simulink model "carsim_ekf_jonathan"  (R2024a)
settings: Solver=VariableStepAuto  StartTime=0.0  StopTime=40  RelTol=1e-3
model workspace (MAT data in the model file):
  Ts = 0.01
  a = 0.9
  b = 0.8
  for_ekf = mamfis
  for_ekf.Name = "for_ekf"
  for_ekf.Type = "mamdani"
  for_ekf.AndMethod = "min"
  for_ekf.OrMethod = "max"
  for_ekf.FuzzyInferenceSystem.LocalImplicationMethod = "min"
  for_ekf.FuzzyInferenceSystem.LocalAggregationMethod = "max"
  for_ekf.FuzzyInferenceSystem.LocalDefuzzificationMethod = "centroid"
  for_ekf.Inputs = fisvar
  for_ekf.Inputs.LocalName = "input1"
  for_ekf.Inputs.Range = [-30 30]
  for_ekf.Inputs.EvalfisData.name = ' '
  for_ekf.Inputs.EvalfisData.range = [-30 30]
  for_ekf.Inputs.EvalfisData.mf(1).name = ' '
  for_ekf.Inputs.EvalfisData.mf(1).type = 'linzmf'
  for_ekf.Inputs.EvalfisData.mf(1).params = [-20 -10]
  for_ekf.Inputs.EvalfisData.mf(2).name = ' '
  for_ekf.Inputs.EvalfisData.mf(2).type = 'trapmf'
  for_ekf.Inputs.EvalfisData.mf(2).params = [-20 -10 10 20]
  for_ekf.Inputs.EvalfisData.mf(3).name = ' '
  for_ekf.Inputs.EvalfisData.mf(3).type = 'linsmf'
  for_ekf.Inputs.EvalfisData.mf(3).params = [10 20]
  for_ekf.Inputs.LocalMembershipFunctions(1) = fismf
  for_ekf.Inputs.LocalMembershipFunctions(1).Function : function handle (value not decoded)
  for_ekf.Inputs.LocalMembershipFunctions(1).Parameters = [-20 -10]
  for_ekf.Inputs.LocalMembershipFunctions(1).ParameterValueValidator : function handle (value not decoded)
  for_ekf.Inputs.LocalMembershipFunctions(1).NumParameters = 2
  for_ekf.Inputs.LocalMembershipFunctions(1).TypeStr = "linzmf"
  for_ekf.Inputs.LocalMembershipFunctions(1).EvalfisData.name = ' '
  for_ekf.Inputs.LocalMembershipFunctions(1).EvalfisData.type = 'linzmf'
  for_ekf.Inputs.LocalMembershipFunctions(1).EvalfisData.params = [-20 -10]
  for_ekf.Inputs.LocalMembershipFunctions(1).fuzzy.internal.fis.MembershipFunction.LocalName = "high1"
  for_ekf.Inputs.LocalMembershipFunctions(1).UnmatchedInputArguments = struct()
  for_ekf.Inputs.LocalMembershipFunctions(2) = fismf
  for_ekf.Inputs.LocalMembershipFunctions(2).Function : function handle (value not decoded)
  for_ekf.Inputs.LocalMembershipFunctions(2).Parameters = [-20 -10 10 20]
  for_ekf.Inputs.LocalMembershipFunctions(2).ParameterValueValidator : function handle (value not decoded)
  for_ekf.Inputs.LocalMembershipFunctions(2).NumParameters = 4
  for_ekf.Inputs.LocalMembershipFunctions(2).TypeStr = "trapmf"
  for_ekf.Inputs.LocalMembershipFunctions(2).EvalfisData.name = ' '
  for_ekf.Inputs.LocalMembershipFunctions(2).EvalfisData.type = 'trapmf'
  for_ekf.Inputs.LocalMembershipFunctions(2).EvalfisData.params = [-20 -10 10 20]
  for_ekf.Inputs.LocalMembershipFunctions(2).fuzzy.internal.fis.MembershipFunction.LocalName = "mf2"
  for_ekf.Inputs.LocalMembershipFunctions(2).UnmatchedInputArguments = struct()
  for_ekf.Inputs.LocalMembershipFunctions(3) = fismf
  for_ekf.Inputs.LocalMembershipFunctions(3).Function : function handle (value not decoded)
  for_ekf.Inputs.LocalMembershipFunctions(3).Parameters = [10 20]
  for_ekf.Inputs.LocalMembershipFunctions(3).ParameterValueValidator : function handle (value not decoded)
  for_ekf.Inputs.LocalMembershipFunctions(3).NumParameters = 2
  for_ekf.Inputs.LocalMembershipFunctions(3).TypeStr = "linsmf"
  for_ekf.Inputs.LocalMembershipFunctions(3).EvalfisData.name = ' '
  for_ekf.Inputs.LocalMembershipFunctions(3).EvalfisData.type = 'linsmf'
  for_ekf.Inputs.LocalMembershipFunctions(3).EvalfisData.params = [10 20]
  for_ekf.Inputs.LocalMembershipFunctions(3).fuzzy.internal.fis.MembershipFunction.LocalName = "high2"
  for_ekf.Inputs.LocalMembershipFunctions(3).UnmatchedInputArguments = struct()
  for_ekf.Outputs = fisvar
  for_ekf.Outputs.LocalName = "output1"
  for_ekf.Outputs.Range = [0 10000]
  for_ekf.Outputs.EvalfisData.name = ' '
  for_ekf.Outputs.EvalfisData.range = [0 10000]
  for_ekf.Outputs.EvalfisData.mf(1).name = ' '
  for_ekf.Outputs.EvalfisData.mf(1).type = 'trimf'
  for_ekf.Outputs.EvalfisData.mf(1).params = [10000 10000 10000]
  for_ekf.Outputs.EvalfisData.mf(2).name = ' '
  for_ekf.Outputs.EvalfisData.mf(2).type = 'trimf'
  for_ekf.Outputs.EvalfisData.mf(2).params = [0 0 0]
  for_ekf.Outputs.LocalMembershipFunctions(1) = fismf
  for_ekf.Outputs.LocalMembershipFunctions(1).Function : function handle (value not decoded)
  for_ekf.Outputs.LocalMembershipFunctions(1).Parameters = [10000 10000 10000]
  for_ekf.Outputs.LocalMembershipFunctions(1).ParameterValueValidator : function handle (value not decoded)
  for_ekf.Outputs.LocalMembershipFunctions(1).NumParameters = 3
  for_ekf.Outputs.LocalMembershipFunctions(1).TypeStr = "trimf"
  for_ekf.Outputs.LocalMembershipFunctions(1).EvalfisData.name = ' '
  for_ekf.Outputs.LocalMembershipFunctions(1).EvalfisData.type = 'trimf'
  for_ekf.Outputs.LocalMembershipFunctions(1).EvalfisData.params = [10000 10000 10000]
  for_ekf.Outputs.LocalMembershipFunctions(1).fuzzy.internal.fis.MembershipFunction.LocalName = "mf1"
  for_ekf.Outputs.LocalMembershipFunctions(1).UnmatchedInputArguments = struct()
  for_ekf.Outputs.LocalMembershipFunctions(2) = fismf
  for_ekf.Outputs.LocalMembershipFunctions(2).Function : function handle (value not decoded)
  for_ekf.Outputs.LocalMembershipFunctions(2).Parameters = [0 0 0]
  for_ekf.Outputs.LocalMembershipFunctions(2).ParameterValueValidator : function handle (value not decoded)
  for_ekf.Outputs.LocalMembershipFunctions(2).NumParameters = 3
  for_ekf.Outputs.LocalMembershipFunctions(2).TypeStr = "trimf"
  for_ekf.Outputs.LocalMembershipFunctions(2).EvalfisData.name = ' '
  for_ekf.Outputs.LocalMembershipFunctions(2).EvalfisData.type = 'trimf'
  for_ekf.Outputs.LocalMembershipFunctions(2).EvalfisData.params = [0 0 0]
  for_ekf.Outputs.LocalMembershipFunctions(2).fuzzy.internal.fis.MembershipFunction.LocalName = "mf2"
  for_ekf.Outputs.LocalMembershipFunctions(2).UnmatchedInputArguments = struct()
  for_ekf.Rules(1) = fisrule
  for_ekf.Rules(1).LocalAntecedent = 1
  for_ekf.Rules(1).LocalConsequent = 1
  for_ekf.Rules(1).LocalDescription.input.name = "input1"
  for_ekf.Rules(1).LocalDescription.input.mf = "high1"
  for_ekf.Rules(1).LocalDescription.input.complement = 0
  for_ekf.Rules(1).LocalDescription.output.name = "output1"
  for_ekf.Rules(1).LocalDescription.output.mf = "mf1"
  for_ekf.Rules(1).LocalDescription.output.complement = 0
  for_ekf.Rules(1).LocalDescription.weight = 1
  for_ekf.Rules(1).LocalDescription.connection = 1
  for_ekf.Rules(1).LocalWeight = 1
  for_ekf.Rules(1).LocalConnection = 1
  for_ekf.Rules(1).EvalfisData.antecedent = 1
  for_ekf.Rules(1).EvalfisData.consequent = 1
  for_ekf.Rules(1).EvalfisData.weight = 1
  for_ekf.Rules(1).EvalfisData.connection = 1
  for_ekf.Rules(2) = fisrule
  for_ekf.Rules(2).LocalAntecedent = 3
  for_ekf.Rules(2).LocalConsequent = 1
  for_ekf.Rules(2).LocalDescription.input.name = "input1"
  for_ekf.Rules(2).LocalDescription.input.mf = "high2"
  for_ekf.Rules(2).LocalDescription.input.complement = 0
  for_ekf.Rules(2).LocalDescription.output.name = "output1"
  for_ekf.Rules(2).LocalDescription.output.mf = "mf1"
  for_ekf.Rules(2).LocalDescription.output.complement = 0
  for_ekf.Rules(2).LocalDescription.weight = 1
  for_ekf.Rules(2).LocalDescription.connection = 1
  for_ekf.Rules(2).LocalWeight = 1
  for_ekf.Rules(2).LocalConnection = 1
  for_ekf.Rules(2).EvalfisData.antecedent = 3
  for_ekf.Rules(2).EvalfisData.consequent = 1
  for_ekf.Rules(2).EvalfisData.weight = 1
  for_ekf.Rules(2).EvalfisData.connection = 1
  for_ekf.Rules(3) = fisrule
  for_ekf.Rules(3).LocalAntecedent = 2
  for_ekf.Rules(3).LocalConsequent = 2
  for_ekf.Rules(3).LocalDescription.input.name = "input1"
  for_ekf.Rules(3).LocalDescription.input.mf = "mf2"
  for_ekf.Rules(3).LocalDescription.input.complement = 0
  for_ekf.Rules(3).LocalDescription.output.name = "output1"
  for_ekf.Rules(3).LocalDescription.output.mf = "mf2"
  for_ekf.Rules(3).LocalDescription.output.complement = 0
  for_ekf.Rules(3).LocalDescription.weight = 1
  for_ekf.Rules(3).LocalDescription.connection = 1
  for_ekf.Rules(3).LocalWeight = 1
  for_ekf.Rules(3).LocalConnection = 1
  for_ekf.Rules(3).EvalfisData.antecedent = 2
  for_ekf.Rules(3).EvalfisData.consequent = 2
  for_ekf.Rules(3).EvalfisData.weight = 1
  for_ekf.Rules(3).EvalfisData.connection = 1
  for_ekf.EvalfisData.name = ' '
  for_ekf.EvalfisData.type = 'mamdani'
  for_ekf.EvalfisData.andMethod = 'min'
  for_ekf.EvalfisData.orMethod = 'max'
  for_ekf.EvalfisData.defuzzMethod = 'centroid'
  for_ekf.EvalfisData.impMethod = 'min'
  for_ekf.EvalfisData.aggMethod = 'max'
  for_ekf.EvalfisData.input.name = ' '
  for_ekf.EvalfisData.input.range = [-30 30]
  for_ekf.EvalfisData.input.mf(1).name = ' '
  for_ekf.EvalfisData.input.mf(1).type = 'linzmf'
  for_ekf.EvalfisData.input.mf(1).params = [-20 -10]
  for_ekf.EvalfisData.input.mf(2).name = ' '
  for_ekf.EvalfisData.input.mf(2).type = 'trapmf'
  for_ekf.EvalfisData.input.mf(2).params = [-20 -10 10 20]
  for_ekf.EvalfisData.input.mf(3).name = ' '
  for_ekf.EvalfisData.input.mf(3).type = 'linsmf'
  for_ekf.EvalfisData.input.mf(3).params = [10 20]
  for_ekf.EvalfisData.output.name = ' '
  for_ekf.EvalfisData.output.range = [0 10000]
  for_ekf.EvalfisData.output.mf(1).name = ' '
  for_ekf.EvalfisData.output.mf(1).type = 'trimf'
  for_ekf.EvalfisData.output.mf(1).params = [10000 10000 10000]
  for_ekf.EvalfisData.output.mf(2).name = ' '
  for_ekf.EvalfisData.output.mf(2).type = 'trimf'
  for_ekf.EvalfisData.output.mf(2).params = [0 0 0]
  for_ekf.EvalfisData.rule(1).antecedent = 1
  for_ekf.EvalfisData.rule(1).consequent = 1
  for_ekf.EvalfisData.rule(1).weight = 1
  for_ekf.EvalfisData.rule(1).connection = 1
  for_ekf.EvalfisData.rule(2).antecedent = 3
  for_ekf.EvalfisData.rule(2).consequent = 1
  for_ekf.EvalfisData.rule(2).weight = 1
  for_ekf.EvalfisData.rule(2).connection = 1
  for_ekf.EvalfisData.rule(3).antecedent = 2
  for_ekf.EvalfisData.rule(3).consequent = 2
  for_ekf.EvalfisData.rule(3).weight = 1
  for_ekf.EvalfisData.rule(3).connection = 1
  theta = 0
  wf = 1.24
  wr = 1.21
libraries: simulink x3, Solver_SF x1, sharedTrackingLibrary x1, dspstat3 x1, fuzblock x1
settings Model: Creator=Jonat  LastModifiedBy=Jonat
settings RTWCC: GPUComputeCapability=3.5

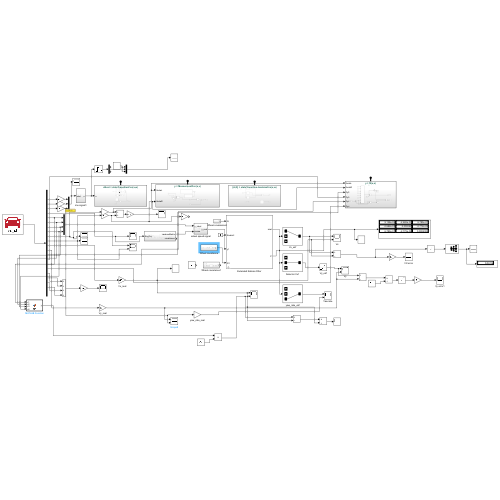
[thumbnail: Simulink's stored preview of the top-level diagram]
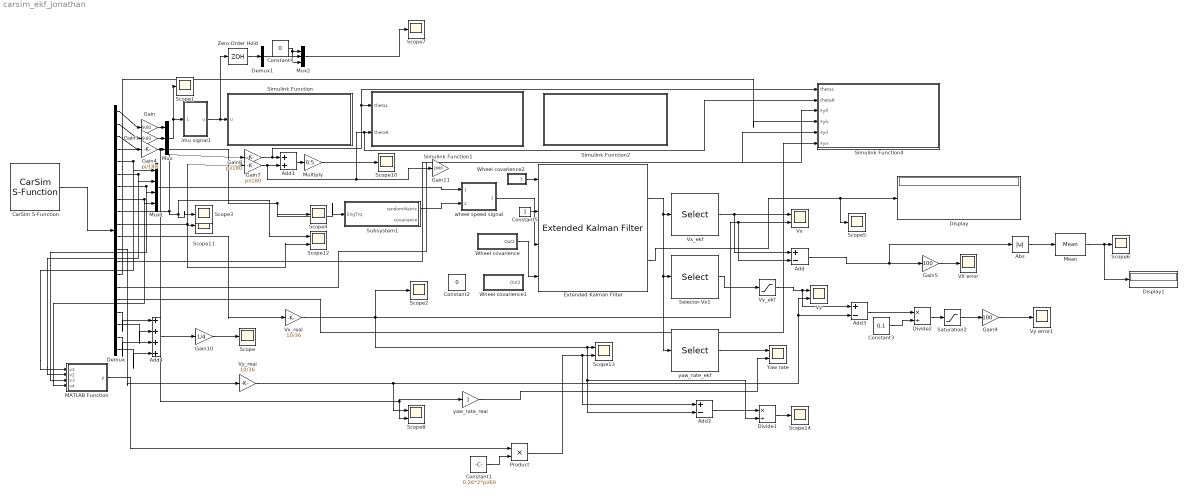
== system carsim_ekf_jonathan ==
  Abs : Abs  SaturateOnIntegerOverflow=off
  Add : Sum  Inputs=+-
  Add1 : Sum
  Add2 : Sum  Inputs=+-
  Add3 : Sum  Inputs=+-
  Add4 : Sum  Inputs=++++
  CarSim S-Function : Solver_SF/CarSim S-Function  Priority=1  SIMFILE=simfile.sim  Run_RTs=off  vs_state_ind=Run  StopMode_ind=Vehicle Model
  Constant1 : Constant  Value=0.26*2*pi/60
  Constant2 : Constant  Value=0
  Constant3 : Constant  Value=0.1
  Constant4 : Constant  Value=0
  Constant5 : Constant
  Demux : Demux  Outputs=20
  Demux1 : Demux  Outputs=3
  Display : Display
  Display1 : Display
  Divide1 : Product  Inputs=*/
  Divide2 : Product  Inputs=*/
  Extended Kalman Filter : sharedTrackingLibrary/Extended Kalman Filter  StateTransitionFcn=stateTransitionFcn  HasStateTransitionJacobianFcn=on  StateTransitionJacobianFcn=stateTransitionJacobianFcn  HasAdditiveProcessNoise=Nonadditive  ProcessNoise=[0.02 0 0;0 0.1 0;0 0 0.0005]  HasTimeVaryingProcessNoise=on  HasStateTransitionFcnExtraArgument=0  InitialState=[15; 0; 0]  InitialStateCovariance=0.0001  MeasurementFcn1=MeasurmentFcn  HasMeasurementJacobianFcn1=off  HasMeasurementEnablePort1=on  HasAdditiveMeasurementNoise1=Nonadditive  MeasurementNoise1=1  HasTimeVaryingMeasurementNoise1=on  HasMeasurementFcnExtraArgument1=0  HasMeasurementWrapping1=off  MeasurementFcn2=f2  HasMeasurementJacobianFcn2=off  HasMeasurementEnablePort2=on  HasAdditiveMeasurementNoise2=Nonadditive  MeasurementNoise2=0.1  HasTimeVaryingMeasurementNoise2=on  HasMeasurementFcnExtraArgument2=0  HasMeasurementWrapping2=off  MeasurementFcn3=myMeasurementFcn  HasMeasurementJacobianFcn3=off  HasMeasurementEnablePort3=off  HasAdditiveMeasurementNoise3=Additive  MeasurementNoise3=1  HasTimeVaryingMeasurementNoise3=off  HasMeasurementFcnExtraArgument3=0  HasMeasurementWrapping3=off  MeasurementFcn4=myMeasurementFcn  HasMeasurementJacobianFcn4=off  HasMeasurementEnablePort4=off  HasAdditiveMeasurementNoise4=Additive  MeasurementNoise4=1  HasTimeVaryingMeasurementNoise4=off  HasMeasurementFcnExtraArgument4=0  HasMeasurementWrapping4=off  MeasurementFcn5=myMeasurementFcn  HasMeasurementJacobianFcn5=off  HasMeasurementEnablePort5=off  HasAdditiveMeasurementNoise5=Additive  MeasurementNoise5=1  HasTimeVaryingMeasurementNoise5=off  HasMeasurementFcnExtraArgument5=0  HasMeasurementWrapping5=off  EnableMultirate=on  StateTransitionFcnSampleTime=0.01  MeasurementFcn1SampleTime=0.01  MeasurementFcn2SampleTime=0.01  MeasurementFcn3SampleTime=1  MeasurementFcn4SampleTime=1  MeasurementFcn5SampleTime=1  UseCurrentEstimator=on  OutputStateCovariance=on  DataType=double  SampleTime=0.01  NumberOfMeasurements=1
      settings: LibrarySourceBlock=slident/Estimators/Extended Kalman Filter
  Gain : Gain  Gain=9.81
  Gain1 : Gain  Gain=9.81
  Gain10 : Gain  Gain=1/4
  Gain11 : Gain  Gain=2000
  Gain4 : Gain  Gain=pi/180
  Gain5 : Gain  Gain=100
  Gain7 : Gain  Gain=pi/180
  Gain8 : Gain  Gain=pi/180
  Gain9 : Gain  Gain=100
  MATLAB Function : MATLAB Function  TreatAsAtomicUnit=on
  Mean : dspstat3/Mean  run=on  InputProcessing=Columns as channels (frame based)  reset_popup=None  directionMode=Each column  dimension=1  roiEnable=off  roiType=Rectangles  roiPortion=Entire ROI  roiOutput=Individual statistics for each ROI  roiFlag=off  roundingMode=Floor  overflowMode=off  outputDataTypeStr=Inherit: Same as accumulator  outputMin=[]  outputMax=[]  outputLastDataTypeStr=Inherit: Same as accumulator
  Multiply : Gain  Gain=0.5
  Mux : Mux  Inputs=3
  Mux1 : Mux
  Mux2 : Mux  Inputs=3
  Product : Product
  Saturation2 : Saturate  UpperLimit=1  LowerLimit=-1
  Scope{,1..7,10..11,14} (11 alike) : Scope
  Scope12 : Scope  NumInputPorts=2
  Scope13 : Scope  NumInputPorts=2
  Scope8 : Scope  NumInputPorts=2
  Selector-Vx1 : Selector  InputPortWidth=3  IndexOptions=Index vector (dialog)  Indices=[2]  OutputSizes=1
  Simulink Function : Subsystem  TreatAsAtomicUnit=on
  Simulink Function1 : Subsystem  TreatAsAtomicUnit=on
  Simulink Function2 : Subsystem  TreatAsAtomicUnit=on
  Simulink Function4 : Subsystem  TreatAsAtomicUnit=on
  Subsystem1 : Subsystem
  VX error : Scope
  Vx : Scope  NumInputPorts=2
  Vx_ekf : Selector  InputPortWidth=3  IndexOptions=Index vector (dialog)  Indices=[1]  OutputSizes=1
  Vx_real : Gain  Gain=10/36
  Vy : Scope  NumInputPorts=2
  Vy error1 : Scope
  Vy_ekf : Saturate  UpperLimit=2  LowerLimit=-2
  Vy_real : Gain  Gain=10/36
  Wheel covarience : Subsystem
  Wheel covarience1 : Subsystem
  Wheel covarience2 : Subsystem
  Yaw rate : Scope  NumInputPorts=2
  Zero-Order Hold : ZeroOrderHold  SampleTime=0.001
  imu signal1 : Subsystem
  wheel speed signal : Subsystem
  yaw_rate_ekf : Selector  InputPortWidth=3  IndexOptions=Index vector (dialog)  Indices=[3]  OutputSizes=1
  yaw_rate_real : Gain
  wires:
  Extended Kalman Filter/1 -> yaw_rate_ekf/1, Selector-Vx1/1, Vx_ekf/1
  wheel speed signal/1(y_real) -> Extended Kalman Filter/3
  Demux/5 -> MATLAB Function/1(v1), Mux1/1
  Demux/6 -> MATLAB Function/2(v2), Mux1/2
  Demux/7 -> MATLAB Function/3(v3), Mux1/3
  Demux/8 -> MATLAB Function/4(v4), Mux1/4
  CarSim S-Function/1 -> Demux/1
  Mux/1 -> imu signal1/1(xdot), Scope1/1
  Mux1/1 -> wheel speed signal/1(y_ideal)
  Demux/4 -> Subsystem1/1(EngTrq), Scope4/1
  Demux/9 -> Scope3/1, Scope12/1, Gain7/1
  Vx_ekf/1 -> Add/1, Vx/1
  Demux/1 -> Gain/1
  Gain/1 -> Mux/1
  Demux/2 -> Gain1/1
  Gain1/1 -> Mux/2
  Demux/11 -> Vx_real/1
  Vx_real/1 -> Scope2/1, Add/2, Vx/2, Add2/2, Divide1/2, Scope13/1
  Multiply/1 -> Scope10/1
  Demux/3 -> Gain4/1
  Gain4/1 -> yaw_rate_real/1, Scope8/2, Mux/3
  imu signal1/1(u) -> Zero-Order Hold/1, Simulink Function/1(u)
  Demux/10 -> Scope12/2, Scope11/1, Gain8/1
  Constant1/1 -> Product/2
  MATLAB Function/1(y) -> Product/1
  Product/1 -> Add2/1, Scope13/2
  Add2/1 -> Divide1/1
  Divide1/1 -> Scope14/1
  Add/1 -> Abs/1, Gain5/1
  Gain5/1 -> VX error/1
  yaw_rate_ekf/1 -> Yaw rate/1
  Add1/1 -> Multiply/1
  Demux/12 -> Vy_real/1
  Selector-Vx1/1 -> Vy_ekf/1
  Gain7/1 -> Simulink Function4/1(thetaL), Simulink Function1/1(thetaL), Add1/1
  Gain8/1 -> Add1/2, Simulink Function4/2(thetaR), Simulink Function1/2(thetaR), Gain11/1
  Saturation2/1 -> Gain9/1
  Gain9/1 -> Vy error1/1
  Divide2/1 -> Saturation2/1
  Vy_real/1 -> Scope8/1, Vy/2, Add3/2
  Add3/1 -> Divide2/1
  Vy_ekf/1 -> Add3/1, Vy/1
  Subsystem1/1(randomMatrix) -> wheel speed signal/2(moise)
  Demux/13 -> Simulink Function4/3(Fyfl)
  Demux/14 -> Simulink Function4/4(Fyfr)
  Demux/15 -> Simulink Function4/5(Fyrl)
  Demux/16 -> Simulink Function4/6(Fyrr)
  Demux/17 -> Add4/1
  Demux/18 -> Add4/2
  Demux/19 -> Add4/3
  Demux/20 -> Add4/4
  Add4/1 -> Gain10/1
  Gain10/1 -> Scope/1
  Constant3/1 -> Divide2/2
  Extended Kalman Filter/2 -> Scope5/1, Display/1
  Zero-Order Hold/1 -> Demux1/1
  Demux1/2 -> Mux2/2
  Constant4/1 -> Mux2/3, Mux2/1
  Mux2/1 -> Scope7/1
  Constant5/1 -> Extended Kalman Filter/2
  Wheel covarience/1(Out2) -> Extended Kalman Filter/4
  yaw_rate_real/1 -> Yaw rate/2
  Mean/1 -> Display1/1, Scope6/1
  Abs/1 -> Mean/1
  Wheel covarience2/1(Out2) -> Extended Kalman Filter/1

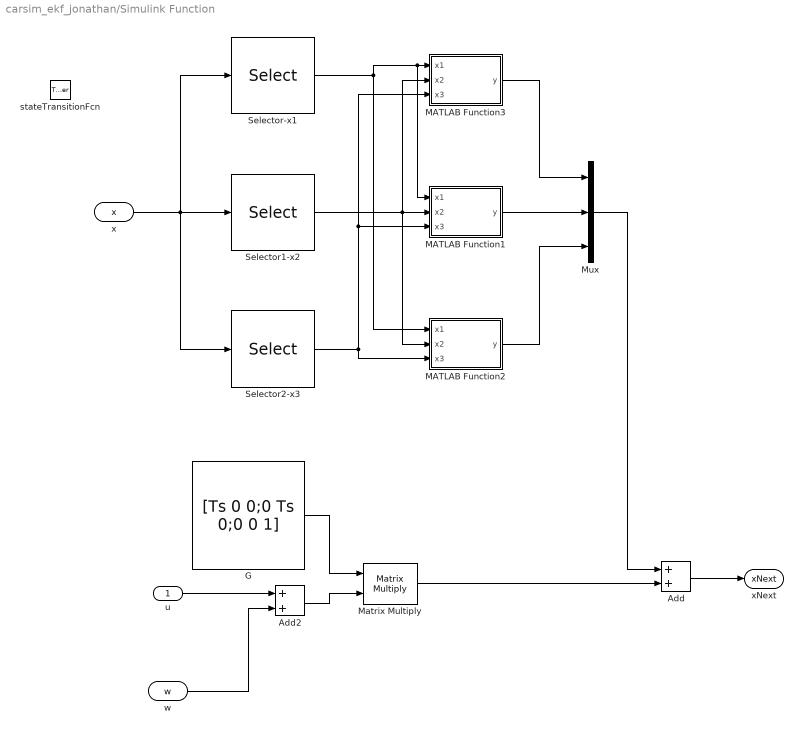
== system carsim_ekf_jonathan/Simulink Function ==
  u : Inport  PortDimensions=3
  stateTransitionFcn : TriggerPort  TriggerType=function-call  IsSimulinkFunction=on  FunctionName=stateTransitionFcn  FunctionVisibility=scoped  VariantControl=(inherit)
  Add : Sum
  Add2 : Sum
  G : Constant  Value=[Ts 0 0;0 Ts 0;0 0 1]
  MATLAB Function1 : MATLAB Function  TreatAsAtomicUnit=on
  MATLAB Function2 : MATLAB Function  TreatAsAtomicUnit=on
  MATLAB Function3 : MATLAB Function  TreatAsAtomicUnit=on
  Matrix Multiply : Product  Multiplication=Matrix(*)
  Mux : Mux  Inputs=3
  Selector-x1 : Selector  InputPortWidth=3  IndexOptions=Index vector (dialog)  Indices=[1]  OutputSizes=1
  Selector1-x2 : Selector  InputPortWidth=3  IndexOptions=Index vector (dialog)  Indices=[2]  OutputSizes=1
  Selector2-x3 : Selector  InputPortWidth=3  IndexOptions=Index vector (dialog)  Indices=[3]  OutputSizes=1
  x : ArgIn  DisableCoverage=on  PortDimensions=3  ArgumentName=x
  w : ArgIn  Port=2  PortDimensions=3  ArgumentName=w
  xNext : ArgOut  DisableCoverage=on  PortDimensions=3  ArgumentName=xNext
  wires:
  x/1 -> Selector2-x3/1, Selector1-x2/1, Selector-x1/1
  Selector-x1/1 -> MATLAB Function2/1(x1), MATLAB Function3/1(x1), MATLAB Function1/1(x1)
  Selector1-x2/1 -> MATLAB Function3/2(x2), MATLAB Function1/2(x2), MATLAB Function2/2(x2)
  Selector2-x3/1 -> MATLAB Function2/3(x3), MATLAB Function3/3(x3), MATLAB Function1/3(x3)
  MATLAB Function3/1(y) -> Mux/1
  MATLAB Function1/1(y) -> Mux/2
  MATLAB Function2/1(y) -> Mux/3
  G/1 -> Matrix Multiply/1
  Matrix Multiply/1 -> Add/2
  Mux/1 -> Add/1
  u/1 -> Add2/1
  Add/1 -> xNext/1
  w/1 -> Add2/2
  Add2/1 -> Matrix Multiply/2

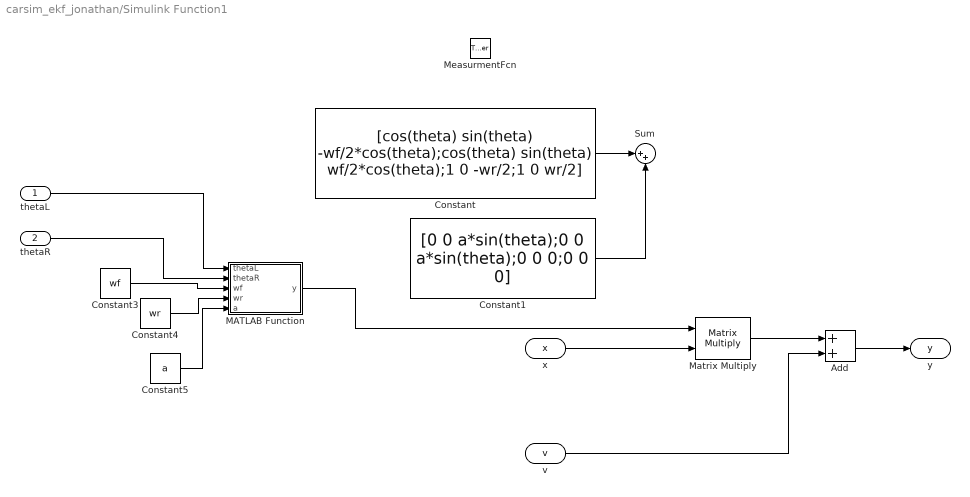
== system carsim_ekf_jonathan/Simulink Function1 ==
  thetaL : Inport
  thetaR : Inport  Port=2
  MeasurmentFcn : TriggerPort  TriggerType=function-call  IsSimulinkFunction=on  FunctionName=MeasurmentFcn  FunctionVisibility=scoped  VariantControl=(inherit)
  Add : Sum
  Constant : Constant  Value=[cos(theta) sin(theta) -wf/2*cos(theta);cos(theta) sin(theta) wf/2*cos(theta);1 0 -wr/2;1 0 wr/2]
  Constant1 : Constant  Value=[0 0 a*sin(theta);0 0 a*sin(theta);0 0 0;0 0 0]
  Constant3 : Constant  Value=wf
  Constant4 : Constant  Value=wr
  Constant5 : Constant  Value=a
  MATLAB Function : MATLAB Function  TreatAsAtomicUnit=on
  Matrix Multiply : Product  Multiplication=Matrix(*)
  Sum : Sum  Inputs=|++
  x : ArgIn  DisableCoverage=on  PortDimensions=3  ArgumentName=x
  v : ArgIn  Port=2  PortDimensions=4  ArgumentName=v
  y : ArgOut  DisableCoverage=on  PortDimensions=4  ArgumentName=y
  wires:
  Constant/1 -> Sum/1
  Constant1/1 -> Sum/2
  x/1 -> Matrix Multiply/2
  Matrix Multiply/1 -> Add/1
  v/1 -> Add/2
  Add/1 -> y/1
  Constant3/1 -> MATLAB Function/3(wf)
  Constant5/1 -> MATLAB Function/5(a)
  thetaL/1 -> MATLAB Function/1(thetaL)
  Constant4/1 -> MATLAB Function/4(wr)
  MATLAB Function/1(y) -> Matrix Multiply/1
  thetaR/1 -> MATLAB Function/2(thetaR)

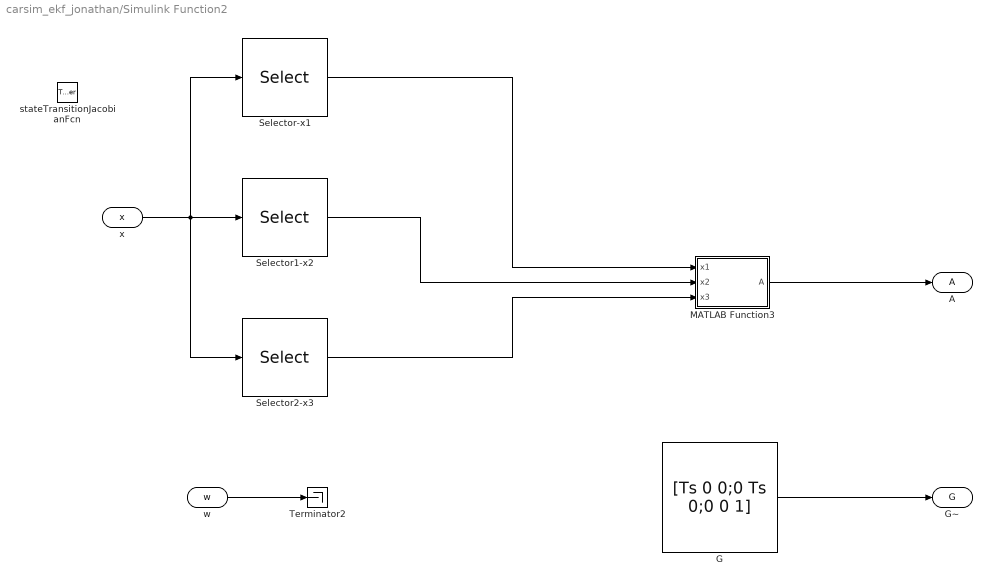
== system carsim_ekf_jonathan/Simulink Function2 ==
  stateTransitionJacobianFcn : TriggerPort  TriggerType=function-call  IsSimulinkFunction=on  FunctionName=stateTransitionJacobianFcn  FunctionVisibility=scoped  VariantControl=(inherit)
  G : Constant  Value=[Ts 0 0;0 Ts 0;0 0 1]
  MATLAB Function3 : MATLAB Function  TreatAsAtomicUnit=on
  Selector-x1 : Selector  InputPortWidth=3  IndexOptions=Index vector (dialog)  Indices=[1]  OutputSizes=1
  Selector1-x2 : Selector  InputPortWidth=3  IndexOptions=Index vector (dialog)  Indices=[2]  OutputSizes=1
  Selector2-x3 : Selector  InputPortWidth=3  IndexOptions=Index vector (dialog)  Indices=[3]  OutputSizes=1
  Terminator2 : Terminator
  x : ArgIn  DisableCoverage=on  PortDimensions=3  ArgumentName=x
  w : ArgIn  Port=2  PortDimensions=3  ArgumentName=w
  A : ArgOut  DisableCoverage=on  PortDimensions=[3 3]  ArgumentName=A
  G~ : ArgOut  Port=2  PortDimensions=[3 3]  ArgumentName=G
  wires:
  x/1 -> Selector2-x3/1, Selector1-x2/1, Selector-x1/1
  w/1 -> Terminator2/1
  G/1 -> G~/1
  Selector-x1/1 -> MATLAB Function3/1(x1)
  Selector1-x2/1 -> MATLAB Function3/2(x2)
  Selector2-x3/1 -> MATLAB Function3/3(x3)
  MATLAB Function3/1(A) -> A/1

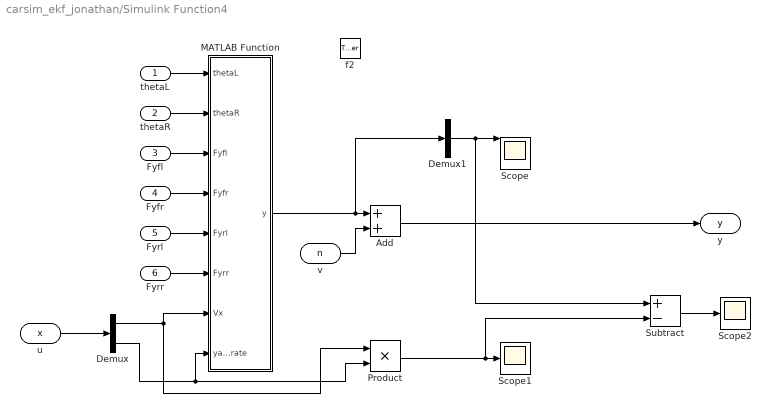
== system carsim_ekf_jonathan/Simulink Function4 ==
  thetaL : Inport
  thetaR : Inport  Port=2
  Fyfl : Inport  Port=3
  Fyfr : Inport  Port=4
  Fyrl : Inport  Port=5
  Fyrr : Inport  Port=6
  f2 : TriggerPort  TriggerType=function-call  IsSimulinkFunction=on  FunctionName=f2  FunctionVisibility=scoped  VariantControl=(inherit)
  Add : Sum
  Demux : Demux  Outputs=3
  Demux1 : Demux  Outputs=3
  MATLAB Function : MATLAB Function  TreatAsAtomicUnit=on
  Product : Product
  Scope : Scope  NumInputPorts=4
  Scope1 : Scope
  Scope2 : Scope
  Subtract : Sum  Inputs=+-
  u : ArgIn  DisableCoverage=on  PortDimensions=3  ArgumentName=x
  v : ArgIn  Port=2  PortDimensions=3  ArgumentName=n
  y : ArgOut  DisableCoverage=on  PortDimensions=3  ArgumentName=y
  wires:
  v/1 -> Add/2
  thetaR/1 -> MATLAB Function/2(thetaR)
  Fyrl/1 -> MATLAB Function/5(Fyrl)
  Add/1 -> y/1
  u/1 -> Demux/1
  Fyrr/1 -> MATLAB Function/6(Fyrr)
  MATLAB Function/1(y) -> Demux1/1, Add/1
  thetaL/1 -> MATLAB Function/1(thetaL)
  Fyfl/1 -> MATLAB Function/3(Fyfl)
  Fyfr/1 -> MATLAB Function/4(Fyfr)
  Demux/1 -> MATLAB Function/7(Vx), Product/1
  Demux/3 -> MATLAB Function/8(yaw_rate), Product/2
  Product/1 -> Subtract/2, Scope1/1
  Demux1/2 -> Subtract/1, Scope/1
  Subtract/1 -> Scope2/1

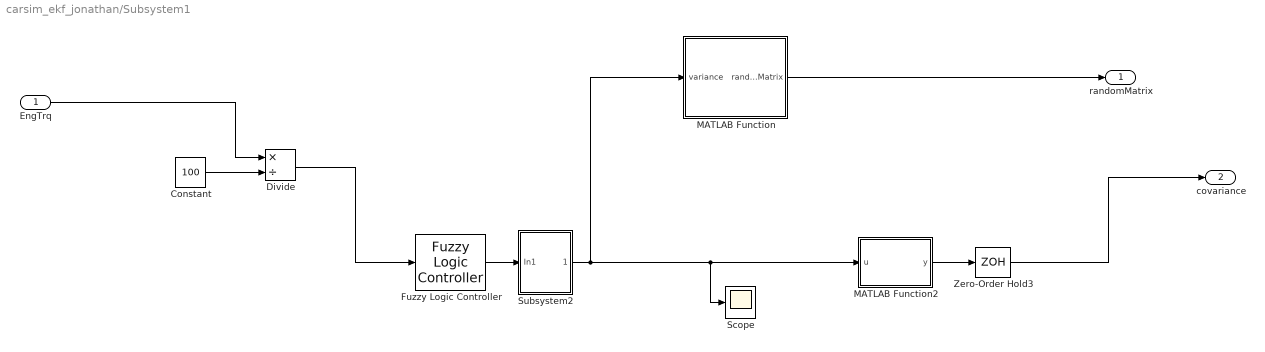
== system carsim_ekf_jonathan/Subsystem1 ==
  EngTrq : Inport
  Constant : Constant  Value=100
  Divide : Product  Inputs=*/
  Fuzzy Logic Controller : fuzblock/Fuzzy Logic  Controller  FIS=for_ekf  OutputSampleNumber=101  DataType=double  FuzzifiedInputs=off  RuleFiringStrengths=off  RuleOutputs=off  AggregatedOutputs=off  SimulateUsing=Interpreted execution  OutOfRangeInputValueMessage=warning  NoRuleFiredMessage=warning  EmptyOutputFuzzySetMessage=warning
  MATLAB Function : MATLAB Function  TreatAsAtomicUnit=on
  MATLAB Function2 : MATLAB Function  TreatAsAtomicUnit=on
  Scope : Scope
  Subsystem2 : Subsystem
  Zero-Order Hold3 : ZeroOrderHold  SampleTime=0.01
  randomMatrix : Outport
  covariance : Outport  Port=2
  wires:
  Subsystem2/1(variance) -> Scope/1, MATLAB Function2/1(u), MATLAB Function/1(variance)
  MATLAB Function2/1(y) -> Zero-Order Hold3/1
  Zero-Order Hold3/1 -> covariance/1
  Constant/1 -> Divide/2
  Fuzzy Logic Controller/1 -> Subsystem2/1(In1)
  Divide/1 -> Fuzzy Logic Controller/1
  EngTrq/1 -> Divide/1
  MATLAB Function/1(randomMatrix) -> randomMatrix/1

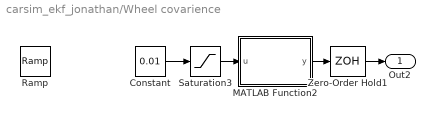
== system carsim_ekf_jonathan/Wheel covarience ==
  Constant : Constant  Value=0.01
  MATLAB Function2 : MATLAB Function  TreatAsAtomicUnit=on
  Ramp : simulink/Sources/Ramp  slope=0.5  start=0  InitialOutput=0.1
  Saturation3 : Saturate  UpperLimit=20
  Zero-Order Hold1 : ZeroOrderHold  SampleTime=0.01
  Out2 : Outport
  wires:
  MATLAB Function2/1(y) -> Zero-Order Hold1/1
  Saturation3/1 -> MATLAB Function2/1(u)
  Zero-Order Hold1/1 -> Out2/1
  Constant/1 -> Saturation3/1

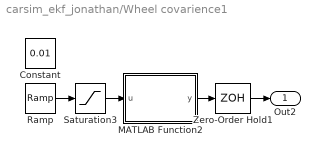
== system carsim_ekf_jonathan/Wheel covarience1 ==
  Constant : Constant  Value=0.01
  MATLAB Function2 : MATLAB Function  TreatAsAtomicUnit=on
  Ramp : simulink/Sources/Ramp  slope=0  start=0  InitialOutput=0.001
  Saturation3 : Saturate  UpperLimit=20
  Zero-Order Hold1 : ZeroOrderHold  SampleTime=0.001
  Out2 : Outport
  wires:
  MATLAB Function2/1(y) -> Zero-Order Hold1/1
  Saturation3/1 -> MATLAB Function2/1(u)
  Ramp/1 -> Saturation3/1
  Zero-Order Hold1/1 -> Out2/1

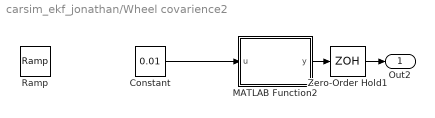
== system carsim_ekf_jonathan/Wheel covarience2 ==
  Constant : Constant  Value=0.01
  MATLAB Function2 : MATLAB Function  TreatAsAtomicUnit=on
  Ramp : simulink/Sources/Ramp  slope=0.5  start=0  InitialOutput=0.1
  Zero-Order Hold1 : ZeroOrderHold  SampleTime=0.01
  Out2 : Outport
  wires:
  MATLAB Function2/1(y) -> Zero-Order Hold1/1
  Constant/1 -> MATLAB Function2/1(u)
  Zero-Order Hold1/1 -> Out2/1

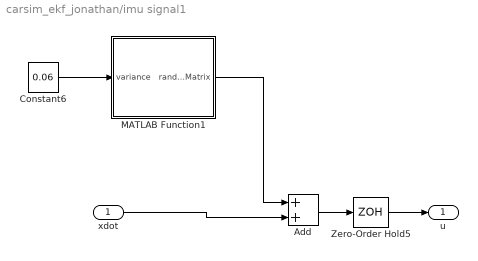
== system carsim_ekf_jonathan/imu signal1 ==
  xdot : Inport
  Add : Sum
  Constant6 : Constant  Value=0.06
  MATLAB Function1 : MATLAB Function  TreatAsAtomicUnit=on
  Zero-Order Hold5 : ZeroOrderHold  SampleTime=0.01
  u : Outport
  wires:
  Zero-Order Hold5/1 -> u/1
  Constant6/1 -> MATLAB Function1/1(variance)
  MATLAB Function1/1(randomMatrix) -> Add/1
  Add/1 -> Zero-Order Hold5/1
  xdot/1 -> Add/2

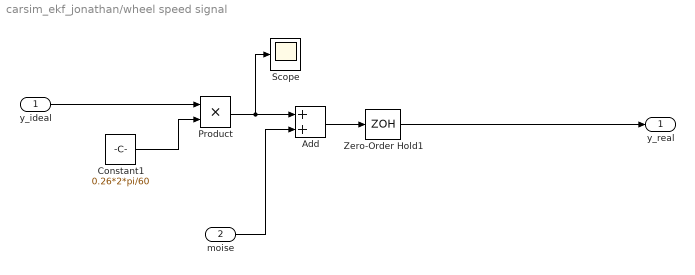
== system carsim_ekf_jonathan/wheel speed signal ==
  y_ideal : Inport
  moise : Inport  Port=2
  Add : Sum
  Constant1 : Constant  Value=0.26*2*pi/60
  Product : Product
  Scope : Scope
  Zero-Order Hold1 : ZeroOrderHold  SampleTime=0.01
  y_real : Outport
  wires:
  Zero-Order Hold1/1 -> y_real/1
  Product/1 -> Add/1, Scope/1
  Constant1/1 -> Product/2
  y_ideal/1 -> Product/1
  Add/1 -> Zero-Order Hold1/1
  moise/1 -> Add/2

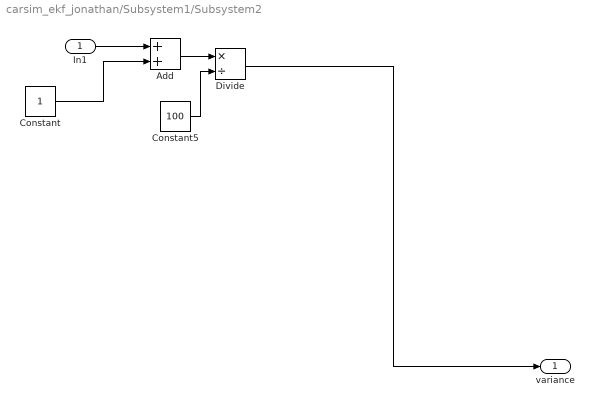
== system carsim_ekf_jonathan/Subsystem1/Subsystem2 ==
  In1 : Inport
  Add : Sum
  Constant : Constant
  Constant5 : Constant  Value=100
  Divide : Product  Inputs=*/
  variance : Outport
  wires:
  Add/1 -> Divide/1
  In1/1 -> Add/1
  Constant5/1 -> Divide/2
  Constant/1 -> Add/2
  Divide/1 -> variance/1

== matlab function carsim_ekf_jonathan/Simulink Function4/MATLAB Function ==
  data: thetaL input; thetaR input; y output; Fyfl input; Fyfr input; Fyrl input; Fyrr input; Vx input; yaw_rate input
function y = fcn(thetaL,thetaR,Fyfl,Fyfr,Fyrl,Fyrr,Vx,yaw_rate)

y = [0; (((Fyfl*cos(thetaL)+Fyfr*cos(thetaR))+(Fyrl+Fyrr))/299.5); 0];

== matlab function carsim_ekf_jonathan/Simulink Function/MATLAB Function3 ==
  data: x1 input; y output; x2 input; x3 input
function y = fcn(x1,x2,x3)

y = x1+0.01*x2*x3;

== matlab function carsim_ekf_jonathan/Wheel covarience2/MATLAB Function2 ==
  data: u input; y output
function y = fcn(u)

y = [u 0 0;
     0 u 0;
     0 0 u];

== matlab function carsim_ekf_jonathan/MATLAB Function ==
  data: v1 input; y output; v2 input; v3 input; v4 input
function y = fcn(v1,v2,v3,v4)

y = (v1+v2+v3+v4)/4;

== matlab function carsim_ekf_jonathan/Wheel covarience1/MATLAB Function2 ==
  data: u input; y output
function y = fcn(u)

y = [u 0 0;
     0 u 0;
     0 0 u];

== matlab function carsim_ekf_jonathan/Subsystem1/MATLAB Function ==
  settings: updateMethod=DISCRETE
  data: variance input; randomMatrix output
function randomMatrix = generateGaussianRandomMatrix(variance)
    % 生成具有高斯分布的4x1矩阵
    % 输入参数：
    %   variance: 方差
    % 输出参数：
    %   randomMatrix: 4x1矩阵

    % 使用 randn 函数生成高斯分布的随机值，并构建4x1矩阵
    randomValues = sqrt(variance) * randn(4, 1);

    % 将随机值存储为4x1矩阵
    randomMatrix = randomValues;
end

== matlab function carsim_ekf_jonathan/Wheel covarience/MATLAB Function2 ==
  data: u input; y output
function y = fcn(u)

y = [u 0 0 0;
     0 u 0 0;
     0 0 u 0;
     0 0 0 u];

== matlab function carsim_ekf_jonathan/Simulink Function/MATLAB Function1 ==
  data: x1 input; y output; x2 input; x3 input
function y = fcn(x1,x2,x3)

y = x2-0.01*x1*x3;

== matlab function carsim_ekf_jonathan/Simulink Function/MATLAB Function2 ==
  data: x1 input; y output; x2 input; x3 input
function y = fcn(x1,x2,x3)

y = 0;

== matlab function carsim_ekf_jonathan/Simulink Function1/MATLAB Function ==
  data: thetaL input; thetaR input; y output; wf input; wr input; a input
function y = fcn(thetaL,thetaR,wf,wr,a)

y = [cos(thetaL) sin(thetaL) (-(wf/2)*cos(thetaL)+a*sin(thetaL)); cos(thetaR) sin(thetaR) ((wf/2)*cos(thetaR)+a*sin(thetaR)); 1 0 -wr/2; 1 0 wr/2];

== matlab function carsim_ekf_jonathan/Simulink Function2/MATLAB Function3 ==
  data: x1 input; A output; x2 input; x3 input
function A = fcn(x1,x2,x3)


Ts=0.01;
A = [1 Ts*x3 Ts*x2; -Ts*x3 1 -Ts*x1; 0 0 0];

== matlab function carsim_ekf_jonathan/imu signal1/MATLAB Function1 ==
  data: variance input; randomMatrix output
function randomMatrix = generateGaussianRandomMatrix(variance)
    % 生成具有高斯分布的4x1矩阵
    % 输入参数：
    %   variance: 方差
    % 输出参数：
    %   randomMatrix: 4x1矩阵

    % 使用 randn 函数生成高斯分布的随机值，并构建4x1矩阵
    randomValues = [sqrt(variance) 0 0;0 sqrt(variance) 0;0 0 sqrt(0.005)] * randn(3, 1);

    % 将随机值存储为4x1矩阵
    randomMatrix = randomValues;
end

== matlab function carsim_ekf_jonathan/Subsystem1/MATLAB Function2 ==
  data: u input; y output
function y = fcn(u)
   
y = [u 0 0 0;
     0 u 0 0;
     0 0 u 0;
     0 0 0 u];
